simulink model "npc_controller"  (R2022a)
settings: Solver=FixedStepDiscrete  StartTime=0.0  StopTime=20  RelTol=1e-3  EnableMultiTasking=on
undefined symbols (not defined in the file): CAN_O_INT, CANA_BASE, Down, GPTRIP1SEL, GPTRIP2SEL, GPTRIP3SEL, Tsw, TZ1, TZ2, TZ3, Up, V2G_en
libraries: simulink x171, hdlsllib x90, c2802xlib x46, c2837xDlib x19, c280xlib x12, canmsglib x9, c2838xlib x8, idelinklib_common x5, c2806xlib x2, slpidlib x2, c28004xlib x2, c281xlib x2
(part 1 of 55)
settings Model: DataDictionary=param.sldd  ExtModeTrigDuration=8  Creator=The MathWorks, Inc.  LastModifiedBy=sgcesuser3
settings SolverCC: AlgebraicLoopSolver=TrustRegion  AutoInsertRateTranBlk=on  MaxZcPerStep=1
settings DataIOCC: LimitDataPoints=on  SaveFormat=Array  SaveOutput=off  SaveTime=off  ReturnWorkspaceOutputs=off
settings OptimizationCC: DefaultParameterBehavior=Inlined  MemcpyThreshold=512  ExpressionDepthLimit=2147483647  LifeSpan=1  MaxStackSize=512  EfficientTunableParamExpr=on
settings DebuggingCC: MergeDetectMultiDrivingBlocksExec=none  SolverPrmCheckMsg=warning  MultiTaskDSMMsg=none  MultiTaskCondExecSysMsg=none  FcnCallInpInsideContextMsg=warning  UnconnectedInputMsg=warning  UnconnectedOutputMsg=warning  UnconnectedLineMsg=warning  AllowSymbolicDim=off  StateNameClashWarn=warning  SFUnexpectedBacktrackingDiag=warning  SFNoUnconditionalDefaultTransitionDiag=warning  SFExecutionAtInitializationDiag=none  SFMachineParentedDataDiag=warning  ArithmeticOperatorsInVariantConditions=warning
settings HardwareCC: ProdBitPerChar=16  ProdBitPerInt=16  ProdBitPerPointer=32  ProdBitPerSizeT=32  ProdBitPerPtrDiffT=32  ProdLargestAtomicInteger=Integer  ProdLargestAtomicFloat=None  ProdWordSize=16  ProdHWDeviceType=Texas Instruments->C2000
settings ModelReferenceCC: ModelReferenceNumInstancesAllowed=Single  PropagateSignalLabelsOutOfModel=off
settings SFSimCC: SimUseLocalCustomCode=off  MATLABDynamicMemAlloc=off  CustomCodeUndefinedFunction=UseInterfaceOnly
settings RTWCC: SystemTargetFile=ert.tlc  HardwareBoard=TI Delfino F2837xS  TemplateMakefile=ert_default_tmf  GenerateReport=on  RTWUseLocalCustomCode=off  Toolchain=Texas Instruments Code Composer Studio (C2000)  BuildConfiguration=Specify  IncludeHyperlinkInReport=on  LaunchReport=on  GenerateTraceInfo=on  GenerateTraceReport=on  GenerateTraceReportSl=on  GenerateTraceReportSf=on  GenerateTraceReportEml=on  DLArmComputeVersion=19.05
settings RTWCC: CustomHeaderCode=|
  | //#include "adc.h"
  | #include "asysctl.h"
  | //#include "can.h"
  | #include "cla.h"
  | #include "cmpss.h"
  | #include "cpu.h"
  | #include "cputimer.h"
  | #include "dac.h"
  | #include "dcsm.h"
  | #include "debug.h"
  | #include "dma.h"
  | #include "ecap.h"
  | #include "emif.h"
  | #include "epwm.h"
  | #include "eqep.h"
  | #include "flash.h"
  | #include "gpio.h"
  | #include "hrpwm.h"
  | #include "i2c.h"
  | #include "interrupt.h"
  | #include "mcbsp.h"
  | #include "memcfg.h"
  | #include "pin_map.h"
  | #include "sci.h"
  | #include "sdfm.h"
  | #include "spi.h"
  | #include "sysctl.h"
  | //#include "upp.h"
  | #include "version.h"
  | #include "xbar.h"
  | //#include "clb.h"
  | //#include "clb_config.h"
settings RTWCC: CustomInclude=|
  | C:\ti\C2000\C2000Ware_4_00_00_00\driverlib\f2837xs\driverlib
  | C:\ti\C2000\C2000Ware_4_00_00_00\device_support\f2837xs\common\include
settings RTWCC: CustomSource=|
  | C:\ti\C2000\C2000Ware_4_00_00_00\driverlib\f2837xs\driverlib\cmpss.c
  | C:\ti\C2000\C2000Ware_4_00_00_00\driverlib\f2837xs\driverlib\xbar.c
  | C:\ti\C2000\C2000Ware_4_00_00_00\driverlib\f2837xs\driverlib\gpio.c
  | C:\ti\C2000\C2000Ware_4_00_00_00\driverlib\f2837xs\driverlib\clb.c
settings CodeAppCC: IgnoreCustomStorageClasses=off  CustomSymbolStrType=$N$R$M  StateflowObjectComments=on  InternalIdentifier=Classic
settings ERTTargetCC: MultiwordLength=2048  ExtModeStaticAllocSize=2048  InlinedParameterPlacement=NonHierarchical  ConvertIfToSwitch=off  SuppressUnreachableDefaultCases=off  MemSecPackage=tic2000demospkg
settings ConfigComp: CovMetricSettings=dw  CovSaveCumulativeToWorkspaceVar=on  CovSaveSingleToWorkspaceVar=on  CovExternalEMLEnable=off  CovSFcnEnable=off

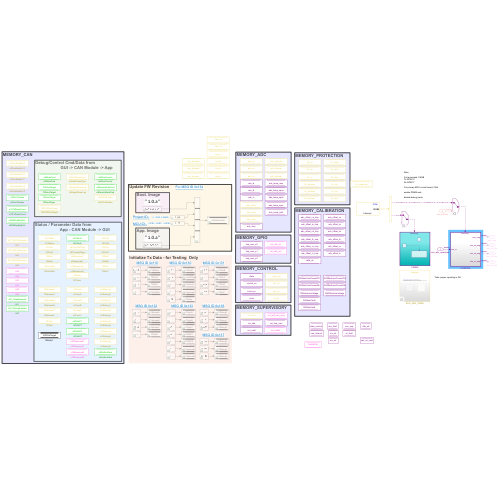
[thumbnail: Simulink's stored preview of the top-level diagram]
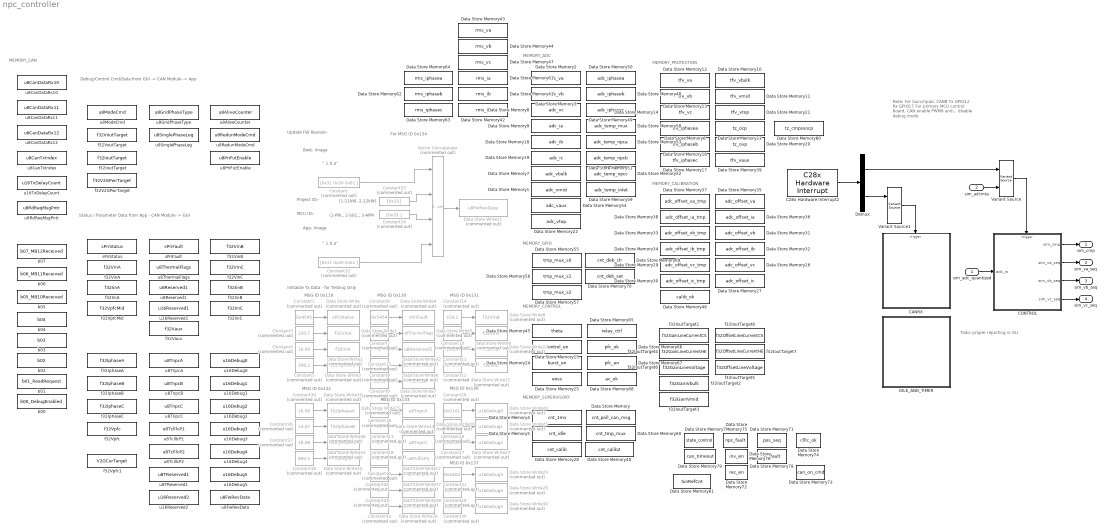
== system npc_controller ==
  note: Todo: proper reporting in GU
  note: MEMORY_CONTROL
  note: MEMORY_ADC
  note: MEMORY_CALIBRATION
  note: MEMORY_GPIO
  note: MEMORY_PROTECTION
  note: MEMORY_SUPERVISORY
  note: Boot. Image
  note: MSG ID 0x110
  note: MSG ID 0x130
  note: " 1.0.a"
  note: For MSG ID 0x134
  note: MSG ID 0x132
  note: Project ID:-
  note: MCU ID:-
  note: MSG ID 0x131
  note: " 1.0.a"
  note: MSG ID 0x133
  note: App. Image
  note: (1-11kW, 2-22kW)
  note: Debug/Control Cmd/Data from
      |                       GUI -> CAN Module -> App
  note: Update FW Revision
  note: Note:
      |
      | For launchpad, CANB
      | Tx GPIO12
      | Rx GPIO17
      |
      | For primary MCU control board, CAN
      |
      | enable PWM9 and...
      |
      | disable debug mode
  note: MEMORY_CAN
  note: Status / Parameter Data from
      |                       App - CAN Module -> GUI
  note: (1-PRI., 2-SEC., 3-APM
  note: MSG ID 0x136
  note: MSG ID 0x137
  note: Initialize Tx Data - for Testing Only
  sim_adc_quantized : Inport
  sim_adcinta : Inport  Port=2  OutputFunctionCall=on
  C28x Hardware Interrupt2 : c2000lib/Scheduling/C28x Hardware Interrupt  irqnumbers=[1 9]  pienumbers=[1 5]  irqpriorities=[30 31]  irqpreempts=[0 1]  showinput=off  dspchiptype=C280X
      settings: SourceProductBaseCode=TIC2000
  CANRX : Subsystem  TreatAsAtomicUnit=on
      settings: RTWFcnNameOpts=Use subsystem name  RTWFileNameOpts=Use subsystem name
  CONTROL : Subsystem  TreatAsAtomicUnit=on  RTWFcnName=Cla1Task1  RTWFileName=sample_cla
      settings: RTWFileNameOpts=User specified  RTWMemSecFuncInitTerm=Default  RTWMemSecFuncExecute=Default  RTWMemSecDataInternal=Default
  Constant : Constant  Commented=on  Value=[0x31 0x30 0x61 ]  OutDataTypeStr=uint8  SampleTime=-1
  Constant1 : Constant  Commented=on  Value=0x4545  OutDataTypeStr=uint16
  Constant10 : Constant  Commented=on  Value=321.2  OutDataTypeStr=single
  Constant11 : Constant  Commented=on  Value=15.09  OutDataTypeStr=single
  Constant12 : Constant  Commented=on  Value=17.09  OutDataTypeStr=single
  Constant13 : Constant  Commented=on  Value=28  OutDataTypeStr=uint8
  Constant14 : Constant  Commented=on  Value=319.2  OutDataTypeStr=single
  Constant16 : Constant  Commented=on  Value=25  OutDataTypeStr=uint8
  Constant17 : Constant  Commented=on  Value=27  OutDataTypeStr=uint8
  Constant18 : Constant  Commented=on  Value=31  OutDataTypeStr=uint8
  Constant26 : Constant  Commented=on  Value=0x0202  OutDataTypeStr=uint16
  Constant27 : Constant  Commented=on  Value=0x0303  OutDataTypeStr=uint16
  Constant28 : Constant  Commented=on  Value=0x0101  OutDataTypeStr=uint16
  Constant29 : Constant  Commented=on  Value=0x0505  OutDataTypeStr=uint16
  Constant3 : Constant  Commented=on  Value=320.7  OutDataTypeStr=single
  Constant30 : Constant  Commented=on  Value=0x0606  OutDataTypeStr=uint16
  Constant31 : Constant  Commented=on  Value=0x0404  OutDataTypeStr=uint16
  Constant32 : Constant  Commented=on  Value=[0x31 0x30 0x61 ]  OutDataTypeStr=uint8  SampleTime=-1
  Constant33 : Constant  Commented=on  Value=[0x31]  OutDataTypeStr=uint8  SampleTime=-1
  Constant34 : Constant  Commented=on  Value=[0x31 ]  OutDataTypeStr=uint8  SampleTime=-1
  Constant35 : Constant  Commented=on  Value=0  OutDataTypeStr=uint8
  Constant36 : Constant  Commented=on  Value=14.07  OutDataTypeStr=single
  Constant37 : Constant  Commented=on  Value=18.08  OutDataTypeStr=single
  Constant38 : Constant  Commented=on  Value=800.5  OutDataTypeStr=single
  Constant39 : Constant  Commented=on  Value=16.09  OutDataTypeStr=single
  Constant4 : Constant  Commented=on  Value=16.09  OutDataTypeStr=single
  Constant40 : Constant  Commented=on  Value=29  OutDataTypeStr=uint8
  Constant41 : Constant  Commented=on  Value=0  OutDataTypeStr=uint8
  Constant42 : Constant  Commented=on  Value=0  OutDataTypeStr=uint16
  Constant5 : Constant  Commented=on  Value=396.2  OutDataTypeStr=single
  Constant6 : Constant  Commented=on  Value=0x5454  OutDataTypeStr=uint16
  Constant7 : Constant  Commented=on  Value=0x0A  OutDataTypeStr=uint8
  Constant8 : Constant  Commented=on  Value=0  OutDataTypeStr=uint16
  Constant9 : Constant  Commented=on  Value=11.95  OutDataTypeStr=single
  Data Store Memory : DataStoreMemory  DataStoreName=cnt_poll_can_msg  ReadBeforeWriteMsg=warning  WriteAfterWriteMsg=warning  WriteAfterReadMsg=warning  ShowAdditionalParam=off  OutDataTypeStr=uint16
  Data Store Memory1 : DataStoreMemory  DataStoreName=adc_vmid  ReadBeforeWriteMsg=warning  WriteAfterWriteMsg=warning  WriteAfterReadMsg=warning  ShowAdditionalParam=off  OutDataTypeStr=single
  Data Store Memory10 : DataStoreMemory  DataStoreName=tfv_vbulk  ReadBeforeWriteMsg=warning  WriteAfterWriteMsg=warning  WriteAfterReadMsg=warning  ShowAdditionalParam=off  OutDataTypeStr=boolean
  Data Store Memory11 : DataStoreMemory  DataStoreName=tfv_vmid  ReadBeforeWriteMsg=warning  WriteAfterWriteMsg=warning  WriteAfterReadMsg=warning  ShowAdditionalParam=off  OutDataTypeStr=boolean
  Data Store Memory12 : DataStoreMemory  DataStoreName=tfv_va  ReadBeforeWriteMsg=warning  WriteAfterWriteMsg=warning  WriteAfterReadMsg=warning  ShowAdditionalParam=off  OutDataTypeStr=boolean
  Data Store Memory13 : DataStoreMemory  DataStoreName=tfv_vb  ReadBeforeWriteMsg=warning  WriteAfterWriteMsg=warning  WriteAfterReadMsg=warning  ShowAdditionalParam=off  OutDataTypeStr=boolean
  Data Store Memory14 : DataStoreMemory  DataStoreName=tfv_vc  ReadBeforeWriteMsg=warning  WriteAfterWriteMsg=warning  WriteAfterReadMsg=warning  ShowAdditionalParam=off  OutDataTypeStr=boolean
  Data Store Memory15 : DataStoreMemory  DataStoreName=control_en  ReadBeforeWriteMsg=warning  WriteAfterWriteMsg=warning  WriteAfterReadMsg=warning  ShowAdditionalParam=off  OutDataTypeStr=boolean
  Data Store Memory16 : DataStoreMemory  DataStoreName=tfv_iphaseb  ReadBeforeWriteMsg=warning  WriteAfterWriteMsg=warning  WriteAfterReadMsg=warning  ShowAdditionalParam=off  OutDataTypeStr=boolean
  Data Store Memory17 : DataStoreMemory  DataStoreName=tfv_iphasec  ReadBeforeWriteMsg=warning  WriteAfterWriteMsg=warning  WriteAfterReadMsg=warning  ShowAdditionalParam=off  OutDataTypeStr=boolean
  Data Store Memory18 : DataStoreMemory  DataStoreName=adc_ib  ReadBeforeWriteMsg=warning  WriteAfterWriteMsg=warning  WriteAfterReadMsg=warning  ShowAdditionalParam=off  OutDataTypeStr=single
  Data Store Memory19 : DataStoreMemory  DataStoreName=adc_ic  ReadBeforeWriteMsg=warning  WriteAfterWriteMsg=warning  WriteAfterReadMsg=warning  ShowAdditionalParam=off  OutDataTypeStr=single
  Data Store Memory2 : DataStoreMemory  DataStoreName=adc_va  ReadBeforeWriteMsg=warning  WriteAfterWriteMsg=warning  WriteAfterReadMsg=warning  ShowAdditionalParam=off  OutDataTypeStr=single
  Data Store Memory20 : DataStoreMemory  DataStoreName=tz_ovp  ReadBeforeWriteMsg=warning  WriteAfterWriteMsg=warning  WriteAfterReadMsg=warning  ShowAdditionalParam=off  OutDataTypeStr=uint16
  Data Store Memory21 : DataStoreMemory  DataStoreName=tfv_vtop  ReadBeforeWriteMsg=warning  WriteAfterWriteMsg=warning  WriteAfterReadMsg=warning  ShowAdditionalParam=off  OutDataTypeStr=boolean
  Data Store Memory22 : DataStoreMemory  DataStoreName=adc_vtop  ReadBeforeWriteMsg=warning  WriteAfterWriteMsg=warning  WriteAfterReadMsg=warning  InitialValue=13  ShowAdditionalParam=off  OutDataTypeStr=uint16
  Data Store Memory23 : DataStoreMemory  DataStoreName=tz_ocp  ReadBeforeWriteMsg=warning  WriteAfterWriteMsg=warning  WriteAfterReadMsg=warning  ShowAdditionalParam=off  OutDataTypeStr=uint16
  Data Store Memory24 : DataStoreMemory  DataStoreName=burst_en  ReadBeforeWriteMsg=warning  WriteAfterWriteMsg=warning  WriteAfterReadMsg=warning  ShowAdditionalParam=off  OutDataTypeStr=boolean
  Data Store Memory25 : DataStoreMemory  DataStoreName=eoss  ReadBeforeWriteMsg=warning  WriteAfterWriteMsg=warning  WriteAfterReadMsg=warning  ShowAdditionalParam=off  OutDataTypeStr=boolean
  Data Store Memory26 : DataStoreMemory  DataStoreName=adc_offset_vc  ReadBeforeWriteMsg=warning  WriteAfterWriteMsg=warning  WriteAfterReadMsg=warning  ShowAdditionalParam=off  OutDataTypeStr=single
  Data Store Memory27 : DataStoreMemory  DataStoreName=adc_offset_ic  ReadBeforeWriteMsg=warning  WriteAfterWriteMsg=warning  WriteAfterReadMsg=warning  ShowAdditionalParam=off  OutDataTypeStr=single
  Data Store Memory28 : DataStoreMemory  DataStoreName=cnt_calib  ReadBeforeWriteMsg=warning  WriteAfterWriteMsg=warning  WriteAfterReadMsg=warning  InitialValue=1  ShowAdditionalParam=off  OutDataTypeStr=uint16
  Data Store Memory29 : DataStoreMemory  DataStoreName=adc_offset_vc_tmp  ReadBeforeWriteMsg=warning  WriteAfterWriteMsg=warning  WriteAfterReadMsg=warning  ShowAdditionalParam=off  OutDataTypeStr=single
  Data Store Memory3 : DataStoreMemory  DataStoreName=adc_vb  ReadBeforeWriteMsg=warning  WriteAfterWriteMsg=warning  WriteAfterReadMsg=warning  ShowAdditionalParam=off  OutDataTypeStr=single
  Data Store Memory30 : DataStoreMemory  DataStoreName=adc_offset_ic_tmp  ReadBeforeWriteMsg=warning  WriteAfterWriteMsg=warning  WriteAfterReadMsg=warning  ShowAdditionalParam=off  OutDataTypeStr=single
  Data Store Memory31 : DataStoreMemory  DataStoreName=adc_offset_vb  ReadBeforeWriteMsg=warning  WriteAfterWriteMsg=warning  WriteAfterReadMsg=warning  ShowAdditionalParam=off  OutDataTypeStr=single
  Data Store Memory32 : DataStoreMemory  DataStoreName=adc_offset_ib  ReadBeforeWriteMsg=warning  WriteAfterWriteMsg=warning  WriteAfterReadMsg=warning  ShowAdditionalParam=off  OutDataTypeStr=single
  Data Store Memory33 : DataStoreMemory  DataStoreName=adc_offset_vb_tmp  ReadBeforeWriteMsg=warning  WriteAfterWriteMsg=warning  WriteAfterReadMsg=warning  ShowAdditionalParam=off  OutDataTypeStr=single
  Data Store Memory34 : DataStoreMemory  DataStoreName=adc_offset_ib_tmp  ReadBeforeWriteMsg=warning  WriteAfterWriteMsg=warning  WriteAfterReadMsg=warning  ShowAdditionalParam=off  OutDataTypeStr=single
  Data Store Memory35 : DataStoreMemory  DataStoreName=adc_offset_va  ReadBeforeWriteMsg=warning  WriteAfterWriteMsg=warning  WriteAfterReadMsg=warning  ShowAdditionalParam=off  OutDataTypeStr=single
  Data Store Memory36 : DataStoreMemory  DataStoreName=adc_offset_ia  ReadBeforeWriteMsg=warning  WriteAfterWriteMsg=warning  WriteAfterReadMsg=warning  ShowAdditionalParam=off  OutDataTypeStr=single
  Data Store Memory37 : DataStoreMemory  DataStoreName=adc_offset_va_tmp  ReadBeforeWriteMsg=warning  WriteAfterWriteMsg=warning  WriteAfterReadMsg=warning  ShowAdditionalParam=off  OutDataTypeStr=single
  Data Store Memory38 : DataStoreMemory  DataStoreName=adc_offset_ia_tmp  ReadBeforeWriteMsg=warning  WriteAfterWriteMsg=warning  WriteAfterReadMsg=warning  ShowAdditionalParam=off  OutDataTypeStr=single
  Data Store Memory39 : DataStoreMemory  DataStoreName=tfv_vaux  ReadBeforeWriteMsg=warning  WriteAfterWriteMsg=warning  WriteAfterReadMsg=warning  ShowAdditionalParam=off  OutDataTypeStr=boolean
  Data Store Memory4 : DataStoreMemory  DataStoreName=cnt_1ms  ReadBeforeWriteMsg=warning  WriteAfterWriteMsg=warning  WriteAfterReadMsg=warning  ShowAdditionalParam=off  OutDataTypeStr=uint16
  Data Store Memory40 : DataStoreMemory  DataStoreName=cnt_calib2  ReadBeforeWriteMsg=warning  WriteAfterWriteMsg=warning  WriteAfterReadMsg=warning  InitialValue=1  ShowAdditionalParam=off  OutDataTypeStr=uint16
  Data Store Memory41 : DataStoreMemory  DataStoreName=rms_ib  ReadBeforeWriteMsg=warning  WriteAfterWriteMsg=warning  WriteAfterReadMsg=warning  ShowAdditionalParam=off  OutDataTypeStr=single
  Data Store Memory42 : DataStoreMemory  DataStoreName=rms_ic  ReadBeforeWriteMsg=warning  WriteAfterWriteMsg=warning  WriteAfterReadMsg=warning  ShowAdditionalParam=off  OutDataTypeStr=single
  Data Store Memory43 : DataStoreMemory  DataStoreName=rms_va  ReadBeforeWriteMsg=warning  WriteAfterWriteMsg=warning  WriteAfterReadMsg=warning  ShowAdditionalParam=off  OutDataTypeStr=single
  Data Store Memory44 : DataStoreMemory  DataStoreName=rms_vb  ReadBeforeWriteMsg=warning  WriteAfterWriteMsg=warning  WriteAfterReadMsg=warning  ShowAdditionalParam=off  OutDataTypeStr=single
  Data Store Memory45 : DataStoreMemory  DataStoreName=theta  ReadBeforeWriteMsg=warning  WriteAfterWriteMsg=warning  WriteAfterReadMsg=warning  ShowAdditionalParam=off  OutDataTypeStr=uint16
  Data Store Memory46 : DataStoreMemory  DataStoreName=calib_ok  ReadBeforeWriteMsg=warning  WriteAfterWriteMsg=warning  WriteAfterReadMsg=warning  ShowAdditionalParam=off  OutDataTypeStr=boolean
  Data Store Memory47 : DataStoreMemory  DataStoreName=rms_vc  ReadBeforeWriteMsg=warning  WriteAfterWriteMsg=warning  WriteAfterReadMsg=warning  ShowAdditionalParam=off  OutDataTypeStr=single
  Data Store Memory48 : DataStoreMemory  DataStoreName=adc_iphaseb  ReadBeforeWriteMsg=warning  WriteAfterWriteMsg=warning  WriteAfterReadMsg=warning  ShowAdditionalParam=off  OutDataTypeStr=single
  Data Store Memory49 : DataStoreMemory  DataStoreName=adc_iphasec  ReadBeforeWriteMsg=warning  WriteAfterWriteMsg=warning  WriteAfterReadMsg=warning  ShowAdditionalParam=off  OutDataTypeStr=single
  Data Store Memory5 : DataStoreMemory  DataStoreName=cnt_idle  ReadBeforeWriteMsg=warning  WriteAfterWriteMsg=warning  WriteAfterReadMsg=warning  ShowAdditionalParam=off  OutDataTypeStr=uint16
  Data Store Memory50 : DataStoreMemory  DataStoreName=adc_iphasea  ReadBeforeWriteMsg=warning  WriteAfterWriteMsg=warning  WriteAfterReadMsg=warning  ShowAdditionalParam=off  OutDataTypeStr=single
  Data Store Memory51 : DataStoreMemory  DataStoreName=adc_temp_npcb  ReadBeforeWriteMsg=warning  WriteAfterWriteMsg=warning  WriteAfterReadMsg=warning  ShowAdditionalParam=off  OutDataTypeStr=single
  Data Store Memory52 : DataStoreMemory  DataStoreName=adc_temp_npcc  ReadBeforeWriteMsg=warning  WriteAfterWriteMsg=warning  WriteAfterReadMsg=warning  ShowAdditionalParam=off  OutDataTypeStr=single
  Data Store Memory53 : DataStoreMemory  DataStoreName=adc_temp_npca  ReadBeforeWriteMsg=warning  WriteAfterWriteMsg=warning  WriteAfterReadMsg=warning  ShowAdditionalParam=off  OutDataTypeStr=single
  Data Store Memory54 : DataStoreMemory  DataStoreName=adc_vaux  ReadBeforeWriteMsg=warning  WriteAfterWriteMsg=warning  WriteAfterReadMsg=warning  ShowAdditionalParam=off  OutDataTypeStr=single
  Data Store Memory55 : DataStoreMemory  DataStoreName=tmp_mux_s0  ReadBeforeWriteMsg=warning  WriteAfterWriteMsg=warning  WriteAfterReadMsg=warning  InitialValue=false  ShowAdditionalParam=off  OutDataTypeStr=boolean
  Data Store Memory56 : DataStoreMemory  DataStoreName=tmp_mux_s1  ReadBeforeWriteMsg=warning  WriteAfterWriteMsg=warning  WriteAfterReadMsg=warning  InitialValue=false  ShowAdditionalParam=off  OutDataTypeStr=boolean
  Data Store Memory57 : DataStoreMemory  DataStoreName=tmp_mux_s2  ReadBeforeWriteMsg=warning  WriteAfterWriteMsg=warning  WriteAfterReadMsg=warning  InitialValue=false  ShowAdditionalParam=off  OutDataTypeStr=boolean
  Data Store Memory58 : DataStoreMemory  DataStoreName=adc_temp_mux  ReadBeforeWriteMsg=warning  WriteAfterWriteMsg=warning  WriteAfterReadMsg=warning  ShowAdditionalParam=off  OutDataTypeStr=single
  Data Store Memory59 : DataStoreMemory  DataStoreName=adc_temp_inlet  ReadBeforeWriteMsg=warning  WriteAfterWriteMsg=warning  WriteAfterReadMsg=warning  ShowAdditionalParam=off  OutDataTypeStr=single
  Data Store Memory6 : DataStoreMemory  DataStoreName=tfv_iphasea  ReadBeforeWriteMsg=warning  WriteAfterWriteMsg=warning  WriteAfterReadMsg=warning  ShowAdditionalParam=off  OutDataTypeStr=boolean
  Data Store Memory60 : DataStoreMemory  DataStoreName=cnt_tmp_mux  ReadBeforeWriteMsg=warning  WriteAfterWriteMsg=warning  WriteAfterReadMsg=warning  ShowAdditionalParam=off  OutDataTypeStr=uint16
  Data Store Memory61 : DataStoreMemory  DataStoreName=rms_ia  ReadBeforeWriteMsg=warning  WriteAfterWriteMsg=warning  WriteAfterReadMsg=warning  ShowAdditionalParam=off  OutDataTypeStr=single
  Data Store Memory62 : DataStoreMemory  DataStoreName=rms_iphaseb  ReadBeforeWriteMsg=warning  WriteAfterWriteMsg=warning  WriteAfterReadMsg=warning  ShowAdditionalParam=off  OutDataTypeStr=single
  Data Store Memory63 : DataStoreMemory  DataStoreName=rms_iphasec  ReadBeforeWriteMsg=warning  WriteAfterWriteMsg=warning  WriteAfterReadMsg=warning  ShowAdditionalParam=off  OutDataTypeStr=single
  Data Store Memory64 : DataStoreMemory  DataStoreName=rms_iphasea  ReadBeforeWriteMsg=warning  WriteAfterWriteMsg=warning  WriteAfterReadMsg=warning  ShowAdditionalParam=off  OutDataTypeStr=single
  Data Store Memory65 : DataStoreMemory  DataStoreName=relay_ctrl  ReadBeforeWriteMsg=warning  WriteAfterWriteMsg=warning  WriteAfterReadMsg=warning  ShowAdditionalParam=off  OutDataTypeStr=boolean
  Data Store Memory66 : DataStoreMemory  DataStoreName=pfc_ok  ReadBeforeWriteMsg=warning  WriteAfterWriteMsg=warning  WriteAfterReadMsg=warning  ShowAdditionalParam=off  OutDataTypeStr=boolean
  Data Store Memory67 : DataStoreMemory  DataStoreName=pfc_en  ReadBeforeWriteMsg=warning  WriteAfterWriteMsg=warning  WriteAfterReadMsg=warning  ShowAdditionalParam=off  OutDataTypeStr=boolean
  Data Store Memory68 : DataStoreMemory  DataStoreName=ac_ok  ReadBeforeWriteMsg=warning  WriteAfterWriteMsg=warning  WriteAfterReadMsg=warning  ShowAdditionalParam=off  OutDataTypeStr=boolean
  Data Store Memory69 : DataStoreMemory  DataStoreName=cnt_deb_clr  WriteAfterWriteMsg=warning  ShowAdditionalParam=off  OutDataTypeStr=uint16
  Data Store Memory7 : DataStoreMemory  DataStoreName=adc_vbulk  ReadBeforeWriteMsg=warning  WriteAfterWriteMsg=warning  WriteAfterReadMsg=warning  ShowAdditionalParam=off  OutDataTypeStr=single
  Data Store Memory70 : DataStoreMemory  DataStoreName=cnt_deb_set  WriteAfterWriteMsg=warning  ShowAdditionalParam=off  OutDataTypeStr=uint16
  Data Store Memory71 : DataStoreMemory  DataStoreName=pos_seq  WriteAfterWriteMsg=warning  ShowAdditionalParam=off
  Data Store Memory72 : DataStoreMemory  DataStoreName=rec_en  WriteAfterWriteMsg=warning  ShowAdditionalParam=off
  Data Store Memory73 : DataStoreMemory  DataStoreName=can_on_cmd  WriteAfterWriteMsg=warning  ShowAdditionalParam=off
  Data Store Memory74 : DataStoreMemory  DataStoreName=clllc_ok  WriteAfterWriteMsg=warning  ShowAdditionalParam=off
  Data Store Memory75 : DataStoreMemory  DataStoreName=npc_fault  WriteAfterWriteMsg=warning  ShowAdditionalParam=off
  Data Store Memory76 : DataStoreMemory  DataStoreName=inv_en  WriteAfterWriteMsg=warning  ShowAdditionalParam=off
  Data Store Memory77 : DataStoreMemory  DataStoreName=state_control  WriteAfterWriteMsg=warning  ShowAdditionalParam=off
  Data Store Memory78 : DataStoreMemory  DataStoreName=ot_fault  WriteAfterWriteMsg=warning  ShowAdditionalParam=off
  Data Store Memory79 : DataStoreMemory  DataStoreName=can_timeout  WriteAfterWriteMsg=warning  ShowAdditionalParam=off
  Data Store Memory8 : DataStoreMemory  DataStoreName=adc_vc  ReadBeforeWriteMsg=warning  WriteAfterWriteMsg=warning  WriteAfterReadMsg=warning  ShowAdditionalParam=off  OutDataTypeStr=single
  Data Store Memory80 : DataStoreMemory  DataStoreName=tz_cmpssocp  ReadBeforeWriteMsg=warning  WriteAfterWriteMsg=warning  WriteAfterReadMsg=warning  ShowAdditionalParam=off  OutDataTypeStr=uint16
  Data Store Memory81 : DataStoreMemory  DataStoreName=SinRefCnt  WriteAfterWriteMsg=warning  ShowAdditionalParam=off  OutDataTypeStr=single
  Data Store Memory9 : DataStoreMemory  DataStoreName=adc_ia  ReadBeforeWriteMsg=warning  WriteAfterWriteMsg=warning  WriteAfterReadMsg=warning  ShowAdditionalParam=off  OutDataTypeStr=single
  Data Store Write : DataStoreWrite  Commented=on  DataStoreName=sPriStatus  IndexOptions=Index vector (dialog)  Indices=1  OutputSizes=1
  Data Store Write1 : DataStoreWrite  Commented=on  DataStoreName=f32VinA  IndexOptions=Index vector (dialog)  Indices=1  OutputSizes=1
  Data Store Write10 : DataStoreWrite  Commented=on  DataStoreName=f32IinB  IndexOptions=Index vector (dialog)  Indices=1  OutputSizes=1
  Data Store Write11 : DataStoreWrite  Commented=on  DataStoreName=f32IinC  IndexOptions=Index vector (dialog)  Indices=1  OutputSizes=1
  Data Store Write14 : DataStoreWrite  Commented=on  DataStoreName=u8TnpcC  IndexOptions=Index vector (dialog)  Indices=1  OutputSizes=1
  Data Store Write15 : DataStoreWrite  Commented=on  DataStoreName=u8TnpcA  IndexOptions=Index vector (dialog)  Indices=1  OutputSizes=1
  Data Store Write16 : DataStoreWrite  Commented=on  DataStoreName=u8TnpcB  IndexOptions=Index vector (dialog)  Indices=1  OutputSizes=1
  Data Store Write17 : DataStoreWrite  Commented=on  DataStoreName=u8TclllcP1  IndexOptions=Index vector (dialog)  Indices=1  OutputSizes=1
  Data Store Write2 : DataStoreWrite  Commented=on  DataStoreName=f32IinA  IndexOptions=Index vector (dialog)  Indices=1  OutputSizes=1
  Data Store Write25 : DataStoreWrite  Commented=on  DataStoreName=u16Debug1  IndexOptions=Index vector (dialog)  Indices=1  OutputSizes=1
  Data Store Write26 : DataStoreWrite  Commented=on  DataStoreName=u16Debug0  IndexOptions=Index vector (dialog)  Indices=1  OutputSizes=1
  Data Store Write27 : DataStoreWrite  Commented=on  DataStoreName=u16Debug2  IndexOptions=Index vector (dialog)  Indices=1  OutputSizes=1
  Data Store Write28 : DataStoreWrite  Commented=on  DataStoreName=u16Debug4  IndexOptions=Index vector (dialog)  Indices=1  OutputSizes=1
  Data Store Write29 : DataStoreWrite  Commented=on  DataStoreName=u16Debug3  IndexOptions=Index vector (dialog)  Indices=1  OutputSizes=1
  Data Store Write3 : DataStoreWrite  Commented=on  DataStoreName=f32VpfcMid  IndexOptions=Index vector (dialog)  Indices=1  OutputSizes=1
  Data Store Write30 : DataStoreWrite  Commented=on  DataStoreName=u16Debug5  IndexOptions=Index vector (dialog)  Indices=1  OutputSizes=1
  Data Store Write31 : DataStoreWrite  Commented=on  DataStoreName=u8FwRevData  IndexOptions=Index vector (dialog)  Indices=1  OutputSizes=1
  Data Store Write32 : DataStoreWrite  Commented=on  DataStoreName=u8Reserved1  IndexOptions=Index vector (dialog)  Indices=1  OutputSizes=1
  Data Store Write33 : DataStoreWrite  Commented=on  DataStoreName=f32IphaseC  IndexOptions=Index vector (dialog)  Indices=1  OutputSizes=1
  Data Store Write34 : DataStoreWrite  Commented=on  DataStoreName=f32Vpfc  IndexOptions=Index vector (dialog)  Indices=1  OutputSizes=1
  Data Store Write35 : DataStoreWrite  Commented=on  DataStoreName=f32IphaseA  IndexOptions=Index vector (dialog)  Indices=1  OutputSizes=1
  Data Store Write36 : DataStoreWrite  Commented=on  DataStoreName=f32IphaseB  IndexOptions=Index vector (dialog)  Indices=1  OutputSizes=1
  Data Store Write37 : DataStoreWrite  Commented=on  DataStoreName=u8TclllcP2  IndexOptions=Index vector (dialog)  Indices=1  OutputSizes=1
  Data Store Write38 : DataStoreWrite  Commented=on  DataStoreName=u8TReserved1  IndexOptions=Index vector (dialog)  Indices=1  OutputSizes=1
  Data Store Write39 : DataStoreWrite  Commented=on  DataStoreName=u16Reserved2  IndexOptions=Index vector (dialog)  Indices=1  OutputSizes=1
  Data Store Write4 : DataStoreWrite  Commented=on  DataStoreName=sPriFault  IndexOptions=Index vector (dialog)  Indices=1  OutputSizes=1
  Data Store Write5 : DataStoreWrite  Commented=on  DataStoreName=u8ThermalFlags  IndexOptions=Index vector (dialog)  Indices=1  OutputSizes=1
  Data Store Write6 : DataStoreWrite  Commented=on  DataStoreName=u16Reserved1  IndexOptions=Index vector (dialog)  Indices=1  OutputSizes=1
  Data Store Write7 : DataStoreWrite  Commented=on  DataStoreName=f32Vaux  IndexOptions=Index vector (dialog)  Indices=1  OutputSizes=1
  Data Store Write8 : DataStoreWrite  Commented=on  DataStoreName=f32VinB  IndexOptions=Index vector (dialog)  Indices=1  OutputSizes=1
  Data Store Write9 : DataStoreWrite  Commented=on  DataStoreName=f32VinC  IndexOptions=Index vector (dialog)  Indices=1  OutputSizes=1
  Demux : Demux  Outputs=2
  IDLE_AND_TIMER : Subsystem  Variant=on
  Variant Source : VariantSource  OutputFunctionCall=on
  Variant Source1 : VariantSource
  Vector Concatenate : Concatenate  Commented=on  NumInputs=4
  b00 : DataStoreMemory  DataStoreName=b00_DebugEnabled  ReadBeforeWriteMsg=warning  WriteAfterWriteMsg=warning  WriteAfterReadMsg=warning  ShowAdditionalParam=off  OutDataTypeStr=boolean
  b01 : DataStoreMemory  DataStoreName=b01_ReadRequest  ReadBeforeWriteMsg=warning  WriteAfterWriteMsg=warning  WriteAfterReadMsg=warning  ShowAdditionalParam=off  OutDataTypeStr=boolean
  b02 : DataStoreMemory  DataStoreName=b02  ReadBeforeWriteMsg=warning  WriteAfterWriteMsg=warning  WriteAfterReadMsg=warning  ShowAdditionalParam=off  OutDataTypeStr=boolean
  b03 : DataStoreMemory  DataStoreName=b03  ReadBeforeWriteMsg=warning  WriteAfterWriteMsg=warning  WriteAfterReadMsg=warning  ShowAdditionalParam=off  OutDataTypeStr=boolean
  b04 : DataStoreMemory  DataStoreName=b04  ReadBeforeWriteMsg=warning  WriteAfterWriteMsg=warning  WriteAfterReadMsg=warning  ShowAdditionalParam=off  OutDataTypeStr=boolean
  b05 : DataStoreMemory  DataStoreName=b05_MB10Received  ReadBeforeWriteMsg=warning  WriteAfterWriteMsg=warning  WriteAfterReadMsg=warning  ShowAdditionalParam=off  OutDataTypeStr=boolean
  b06 : DataStoreMemory  DataStoreName=b06_MB11Received  ReadBeforeWriteMsg=warning  WriteAfterWriteMsg=warning  WriteAfterReadMsg=warning  ShowAdditionalParam=off  OutDataTypeStr=boolean
  b07 : DataStoreMemory  DataStoreName=b07_MB12Received  ReadBeforeWriteMsg=warning  WriteAfterWriteMsg=warning  WriteAfterReadMsg=warning  ShowAdditionalParam=off  OutDataTypeStr=boolean
  f32IinA : DataStoreMemory  DataStoreName=f32IinA  ReadBeforeWriteMsg=warning  WriteAfterWriteMsg=warning  WriteAfterReadMsg=warning  ShowAdditionalParam=off  OutDataTypeStr=single
  f32IinB : DataStoreMemory  DataStoreName=f32IinB  ReadBeforeWriteMsg=warning  WriteAfterWriteMsg=warning  WriteAfterReadMsg=warning  ShowAdditionalParam=off  OutDataTypeStr=single
  f32IinC : DataStoreMemory  DataStoreName=f32IinC  ReadBeforeWriteMsg=warning  WriteAfterWriteMsg=warning  WriteAfterReadMsg=warning  ShowAdditionalParam=off  OutDataTypeStr=single
  f32IoutTarget : DataStoreMemory  DataStoreName=f32IoutTarget  ReadBeforeWriteMsg=warning  WriteAfterWriteMsg=warning  WriteAfterReadMsg=warning  InitialValue=0.0  ShowAdditionalParam=off  OutDataTypeStr=single
  f32IoutTarget1 : DataStoreMemory  DataStoreName=f32GainLineCurrentCS  ReadBeforeWriteMsg=warning  WriteAfterWriteMsg=warning  WriteAfterReadMsg=warning  InitialValue=(3.3/4095)*(1/0.019523)  ShowAdditionalParam=off  OutDataTypeStr=single
  f32IoutTarget2 : DataStoreMemory  DataStoreName=f32GainVbulk  ReadBeforeWriteMsg=warning  WriteAfterWriteMsg=warning  WriteAfterReadMsg=warning  InitialValue=(3.3/4095)*(1/0.00356)  ShowAdditionalParam=off  OutDataTypeStr=single
  f32IoutTarget3 : DataStoreMemory  DataStoreName=f32GainVmid  ReadBeforeWriteMsg=warning  WriteAfterWriteMsg=warning  WriteAfterReadMsg=warning  InitialValue=(3.3/4095)*(1/0.00633)  ShowAdditionalParam=off  OutDataTypeStr=single
  f32IoutTarget4 : DataStoreMemory  DataStoreName=f32GainLineCurrentHE  ReadBeforeWriteMsg=warning  WriteAfterWriteMsg=warning  WriteAfterReadMsg=warning  InitialValue=(3.3/4095)*(1/0.02)  ShowAdditionalParam=off  OutDataTypeStr=single
  f32IoutTarget5 : DataStoreMemory  DataStoreName=f32OffsetLineVoltage  ReadBeforeWriteMsg=warning  WriteAfterWriteMsg=warning  WriteAfterReadMsg=warning  ShowAdditionalParam=off  OutDataTypeStr=single
  f32IoutTarget6 : DataStoreMemory  DataStoreName=f32GainLineVoltage  ReadBeforeWriteMsg=warning  WriteAfterWriteMsg=warning  WriteAfterReadMsg=warning  InitialValue=(3.3/4095)*(1/0.001799)  ShowAdditionalParam=off  OutDataTypeStr=single
  f32IoutTarget7 : DataStoreMemory  DataStoreName=f32OffsetLineCurrentHE  ReadBeforeWriteMsg=warning  WriteAfterWriteMsg=warning  WriteAfterReadMsg=warning  ShowAdditionalParam=off  OutDataTypeStr=single
  f32IoutTarget8 : DataStoreMemory  DataStoreName=f32OffsetLineCurrentCS  ReadBeforeWriteMsg=warning  WriteAfterWriteMsg=warning  WriteAfterReadMsg=warning  ShowAdditionalParam=off  OutDataTypeStr=single
  f32IphaseA : DataStoreMemory  DataStoreName=f32IphaseA  ReadBeforeWriteMsg=warning  WriteAfterWriteMsg=warning  WriteAfterReadMsg=warning  ShowAdditionalParam=off  OutDataTypeStr=single
  f32IphaseB : DataStoreMemory  DataStoreName=f32IphaseB  ReadBeforeWriteMsg=warning  WriteAfterWriteMsg=warning  WriteAfterReadMsg=warning  ShowAdditionalParam=off  OutDataTypeStr=single
  f32IphaseC : DataStoreMemory  DataStoreName=f32IphaseC  ReadBeforeWriteMsg=warning  WriteAfterWriteMsg=warning  WriteAfterReadMsg=warning  ShowAdditionalParam=off  OutDataTypeStr=single
  f32V2GPwrTarget : DataStoreMemory  DataStoreName=f32V2GPwrTarget  ReadBeforeWriteMsg=warning  WriteAfterWriteMsg=warning  WriteAfterReadMsg=warning  InitialValue=0.0  ShowAdditionalParam=off  OutDataTypeStr=single
  f32Vaux : DataStoreMemory  DataStoreName=f32Vaux  ReadBeforeWriteMsg=warning  WriteAfterWriteMsg=warning  WriteAfterReadMsg=warning  ShowAdditionalParam=off  OutDataTypeStr=single
  f32VinA : DataStoreMemory  DataStoreName=f32VinA  ReadBeforeWriteMsg=warning  WriteAfterWriteMsg=warning  WriteAfterReadMsg=warning  ShowAdditionalParam=off  OutDataTypeStr=single
  f32VinB : DataStoreMemory  DataStoreName=f32VinB  ReadBeforeWriteMsg=warning  WriteAfterWriteMsg=warning  WriteAfterReadMsg=warning  ShowAdditionalParam=off  OutDataTypeStr=single
  f32VinC : DataStoreMemory  DataStoreName=f32VinC  ReadBeforeWriteMsg=warning  WriteAfterWriteMsg=warning  WriteAfterReadMsg=warning  ShowAdditionalParam=off  OutDataTypeStr=single
  f32VoutTarget : DataStoreMemory  DataStoreName=f32VoutTarget  ReadBeforeWriteMsg=warning  WriteAfterWriteMsg=warning  WriteAfterReadMsg=warning  InitialValue=0.0  ShowAdditionalParam=off  OutDataTypeStr=single
  f32Vpfc : DataStoreMemory  DataStoreName=f32Vpfc  ReadBeforeWriteMsg=warning  WriteAfterWriteMsg=warning  WriteAfterReadMsg=warning  ShowAdditionalParam=off  OutDataTypeStr=single
  f32Vpfc1 : DataStoreMemory  DataStoreName=V2GCurTarget  ReadBeforeWriteMsg=warning  WriteAfterWriteMsg=warning  WriteAfterReadMsg=warning  ShowAdditionalParam=off  OutDataTypeStr=single
  f32VpfcMid : DataStoreMemory  DataStoreName=f32VpfcMid  ReadBeforeWriteMsg=warning  WriteAfterWriteMsg=warning  WriteAfterReadMsg=warning  ShowAdditionalParam=off  OutDataTypeStr=single
  sPriFault : DataStoreMemory  DataStoreName=sPriFault  ReadBeforeWriteMsg=warning  WriteAfterWriteMsg=warning  WriteAfterReadMsg=warning  ShowAdditionalParam=off  OutDataTypeStr=uint16
  sPriStatus : DataStoreMemory  DataStoreName=sPriStatus  ReadBeforeWriteMsg=warning  WriteAfterWriteMsg=warning  WriteAfterReadMsg=warning  ShowAdditionalParam=off  OutDataTypeStr=uint16
  u16Debug0 : DataStoreMemory  DataStoreName=u16Debug0  ReadBeforeWriteMsg=warning  WriteAfterWriteMsg=warning  WriteAfterReadMsg=warning  ShowAdditionalParam=off  OutDataTypeStr=uint16
  u16Debug1 : DataStoreMemory  DataStoreName=u16Debug1  ReadBeforeWriteMsg=warning  WriteAfterWriteMsg=warning  WriteAfterReadMsg=warning  ShowAdditionalParam=off  OutDataTypeStr=uint16
  u16Debug2 : DataStoreMemory  DataStoreName=u16Debug2  ReadBeforeWriteMsg=warning  WriteAfterWriteMsg=warning  WriteAfterReadMsg=warning  ShowAdditionalParam=off  OutDataTypeStr=uint16
  u16Debug3 : DataStoreMemory  DataStoreName=u16Debug3  ReadBeforeWriteMsg=warning  WriteAfterWriteMsg=warning  WriteAfterReadMsg=warning  ShowAdditionalParam=off  OutDataTypeStr=uint16
  u16Debug4 : DataStoreMemory  DataStoreName=u16Debug4  ReadBeforeWriteMsg=warning  WriteAfterWriteMsg=warning  WriteAfterReadMsg=warning  ShowAdditionalParam=off  OutDataTypeStr=uint16
  u16Debug5 : DataStoreMemory  DataStoreName=u16Debug5  ReadBeforeWriteMsg=warning  WriteAfterWriteMsg=warning  WriteAfterReadMsg=warning  ShowAdditionalParam=off  OutDataTypeStr=uint16
  u16Reserved1 : DataStoreMemory  DataStoreName=u16Reserved1  ReadBeforeWriteMsg=warning  WriteAfterWriteMsg=warning  WriteAfterReadMsg=warning  ShowAdditionalParam=off  OutDataTypeStr=uint16
  u16Reserved2 : DataStoreMemory  DataStoreName=u16Reserved2  ReadBeforeWriteMsg=warning  WriteAfterWriteMsg=warning  WriteAfterReadMsg=warning  ShowAdditionalParam=off  OutDataTypeStr=uint16
  u16TxDelayCount : DataStoreMemory  DataStoreName=u16TxDelayCount  ReadBeforeWriteMsg=warning  WriteAfterWriteMsg=warning  WriteAfterReadMsg=warning  ShowAdditionalParam=off  OutDataTypeStr=uint16
  u8AliveCounter : DataStoreMemory  DataStoreName=u8AliveCounter  ReadBeforeWriteMsg=warning  WriteAfterWriteMsg=warning  WriteAfterReadMsg=warning  ShowAdditionalParam=off  OutDataTypeStr=uint8
  u8CanDataRx10 : DataStoreMemory  DataStoreName=u8CanDataRx10  ReadBeforeWriteMsg=warning  WriteAfterWriteMsg=warning  WriteAfterReadMsg=warning  InitialValue=[0 0 0 0 0 0 0 0]  ShowAdditionalParam=off  OutDataTypeStr=uint8  Dimensions=[8 1]
  u8CanDataRx11 : DataStoreMemory  DataStoreName=u8CanDataRx11  ReadBeforeWriteMsg=warning  WriteAfterWriteMsg=warning  WriteAfterReadMsg=warning  InitialValue=[0 0 0 0 0 0 0 0]  ShowAdditionalParam=off  OutDataTypeStr=uint8  Dimensions=[8 1]
  u8CanDataRx12 : DataStoreMemory  DataStoreName=u8CanDataRx12  ReadBeforeWriteMsg=warning  WriteAfterWriteMsg=warning  WriteAfterReadMsg=warning  InitialValue=[0 0 0 0 0 0 0 0]  ShowAdditionalParam=off  OutDataTypeStr=uint8  Dimensions=[8 1]
  u8CanTxIndex : DataStoreMemory  DataStoreName=u8CanTxIndex  ReadBeforeWriteMsg=warning  WriteAfterWriteMsg=warning  WriteAfterReadMsg=warning  ShowAdditionalParam=off  OutDataTypeStr=uint8
  u8FwRevData : DataStoreMemory  DataStoreName=u8FwRevData  ReadBeforeWriteMsg=warning  WriteAfterWriteMsg=warning  WriteAfterReadMsg=warning  InitialValue=[0 0 0 0 0 0 0 0]  ShowAdditionalParam=off  OutDataTypeStr=uint8  Dimensions=[8 1]
  u8GridPhaseType : DataStoreMemory  DataStoreName=u8GridPhaseType  ReadBeforeWriteMsg=warning  WriteAfterWriteMsg=warning  WriteAfterReadMsg=warning  ShowAdditionalParam=off  OutDataTypeStr=uint8
  u8ModeCmd : DataStoreMemory  DataStoreName=u8ModeCmd  ReadBeforeWriteMsg=warning  WriteAfterWriteMsg=warning  WriteAfterReadMsg=warning  ShowAdditionalParam=off  OutDataTypeStr=uint8
  u8PriFutEnable : DataStoreMemory  DataStoreName=u8PriFutEnable  ReadBeforeWriteMsg=warning  WriteAfterWriteMsg=warning  WriteAfterReadMsg=warning  ShowAdditionalParam=off  OutDataTypeStr=uint8
  u8RdReqMsgPntr : DataStoreMemory  DataStoreName=u8RdReqMsgPntr  ReadBeforeWriteMsg=warning  WriteAfterWriteMsg=warning  WriteAfterReadMsg=warning  ShowAdditionalParam=off  OutDataTypeStr=uint8
  u8RedunModeCmd : DataStoreMemory  DataStoreName=u8RedunModeCmd  ReadBeforeWriteMsg=warning  WriteAfterWriteMsg=warning  WriteAfterReadMsg=warning  ShowAdditionalParam=off  OutDataTypeStr=uint8
  u8Reserved1 : DataStoreMemory  DataStoreName=u8Reserved1  ReadBeforeWriteMsg=warning  WriteAfterWriteMsg=warning  WriteAfterReadMsg=warning  ShowAdditionalParam=off  OutDataTypeStr=uint8
  u8SinglePhaseLeg : DataStoreMemory  DataStoreName=u8SinglePhaseLeg  ReadBeforeWriteMsg=warning  WriteAfterWriteMsg=warning  WriteAfterReadMsg=warning  ShowAdditionalParam=off  OutDataTypeStr=uint8
  u8TReserved1 : DataStoreMemory  DataStoreName=u8TReserved1  ReadBeforeWriteMsg=warning  WriteAfterWriteMsg=warning  WriteAfterReadMsg=warning  ShowAdditionalParam=off  OutDataTypeStr=uint8
  u8TclllcP1 : DataStoreMemory  DataStoreName=u8TclllcP1  ReadBeforeWriteMsg=warning  WriteAfterWriteMsg=warning  WriteAfterReadMsg=warning  ShowAdditionalParam=off  OutDataTypeStr=uint8
  u8TclllcP2 : DataStoreMemory  DataStoreName=u8TclllcP2  ReadBeforeWriteMsg=warning  WriteAfterWriteMsg=warning  WriteAfterReadMsg=warning  ShowAdditionalParam=off  OutDataTypeStr=uint8
  u8ThermalFlags : DataStoreMemory  DataStoreName=u8ThermalFlags  ReadBeforeWriteMsg=warning  WriteAfterWriteMsg=warning  WriteAfterReadMsg=warning  ShowAdditionalParam=off  OutDataTypeStr=uint8
  u8TnpcA : DataStoreMemory  DataStoreName=u8TnpcA  ReadBeforeWriteMsg=warning  WriteAfterWriteMsg=warning  WriteAfterReadMsg=warning  ShowAdditionalParam=off  OutDataTypeStr=uint8
  u8TnpcB : DataStoreMemory  DataStoreName=u8TnpcB  ReadBeforeWriteMsg=warning  WriteAfterWriteMsg=warning  WriteAfterReadMsg=warning  ShowAdditionalParam=off  OutDataTypeStr=uint8
  u8TnpcC : DataStoreMemory  DataStoreName=u8TnpcC  ReadBeforeWriteMsg=warning  WriteAfterWriteMsg=warning  WriteAfterReadMsg=warning  ShowAdditionalParam=off  OutDataTypeStr=uint8
  sim_cmp : Outport
  sim_va_seq : Outport  Port=2
  sim_vb_seq : Outport  Port=3
  sim_vc_seq : Outport  Port=4
  wires:
  sim_adc_quantized/1 -> CONTROL/1(adc_in)
  Demux/1 -> Variant Source/1
  CONTROL/1(sim_cmp) -> sim_cmp/1
  CONTROL/4(sim_vc_seq) -> sim_vc_seq/1
  CONTROL/2(sim_va_seq) -> sim_va_seq/1
  sim_adcinta/1 -> Variant Source/2
  Variant Source/1 -> CONTROL/Trigger
  CONTROL/3(sim_vb_seq) -> sim_vb_seq/1
  C28x Hardware Interrupt2/1 -> Demux/1
  Variant Source1/1 -> CANRX/Trigger
  Demux/2 -> Variant Source1/1
  Constant32/1 -> Vector Concatenate/4
  Constant1/1 -> Data Store Write/1
  Constant28/1 -> Data Store Write26/1
  Vector Concatenate/1 -> Data Store Write31/1
  Constant6/1 -> Data Store Write4/1
  Constant9/1 -> Data Store Write7/1
  Constant38/1 -> Data Store Write34/1
  Constant27/1 -> Data Store Write27/1
  Constant/1 -> Vector Concatenate/1
  Constant17/1 -> Data Store Write17/1
  Constant42/1 -> Data Store Write39/1
  Constant33/1 -> Vector Concatenate/2
  Constant4/1 -> Data Store Write2/1
  Constant12/1 -> Data Store Write11/1
  Constant26/1 -> Data Store Write25/1
  Constant40/1 -> Data Store Write37/1
  Constant35/1 -> Data Store Write32/1
  Constant3/1 -> Data Store Write1/1
  Constant29/1 -> Data Store Write28/1
  Constant18/1 -> Data Store Write14/1
  Constant36/1 -> Data Store Write36/1
  Constant14/1 -> Data Store Write8/1
  Constant41/1 -> Data Store Write38/1
  Constant31/1 -> Data Store Write29/1
  Constant5/1 -> Data Store Write3/1
  Constant11/1 -> Data Store Write10/1
  Constant37/1 -> Data Store Write33/1
  Constant16/1 -> Data Store Write15/1
  Constant13/1 -> Data Store Write16/1
  Constant39/1 -> Data Store Write35/1
  Constant8/1 -> Data Store Write6/1
  Constant34/1 -> Vector Concatenate/3
  Constant7/1 -> Data Store Write5/1
  Constant30/1 -> Data Store Write30/1
  Constant10/1 -> Data Store Write9/1

== system npc_controller/CANRX ==
  function : TriggerPort  TriggerType=function-call  VariantControl=Variant
  Function-Call Generator2 : simulink/Ports & Subsystems/Function-Call Generator  sample_time=-1  numberOfIterations=1  DisallowWideOutput=off
  can_rcv : Subsystem  TreatAsAtomicUnit=on
  wires:
  Function-Call Generator2/1 -> can_rcv/Trigger

== system npc_controller/CONTROL ==
  adc_in : Inport
  function : TriggerPort  TriggerType=function-call  VariantControl=Variant  PortDimensions=1
  CONTROL : Subsystem  TreatAsAtomicUnit=on
      settings: RTWSystemCode=Inline
  Constant : Constant  Commented=on  Value=V2G_en  OutDataTypeStr=single  SampleTime=-1
  Data Store Read : DataStoreRead  DataStoreName=control_en  IndexOptions=Index vector (dialog)  Indices=1  OutputSizes=1
  Data Store Read1 : DataStoreRead  DataStoreName=V2GCurTarget  IndexOptions=Index vector (dialog)  Indices=1  OutputSizes=1
  Data Store Write : DataStoreWrite  DataStoreName=control_en  IndexOptions=Index vector (dialog)  Indices=1  OutputSizes=1
  Data Store Write1 : DataStoreWrite  DataStoreName=burst_en  IndexOptions=Index vector (dialog)  Indices=1  OutputSizes=1
  Data Store Write2 : DataStoreWrite  DataStoreName=eoss  IndexOptions=Index vector (dialog)  Indices=1  OutputSizes=1
  Data Store Write3 : DataStoreWrite  DataStoreName=calib_ok  IndexOptions=Index vector (dialog)  Indices=1  OutputSizes=1
  Function-Call Generator : simulink/Ports & Subsystems/Function-Call Generator  sample_time=-1  numberOfIterations=1  DisallowWideOutput=off
  Function-Call Split{,1..4} (5 alike) : FunctionCallSplit  NumOutputPorts=2
  GET_ADC : Subsystem  TreatAsAtomicUnit=on  RTWFcnName=Cla1Task1  RTWFileName=sample_cla
      settings: RTWSystemCode=Inline  RTWFileNameOpts=User specified  RTWMemSecFuncInitTerm=Default  RTWMemSecFuncExecute=CpuToCla1MsgRAM  RTWMemSecDataInternal=Default
  GPIO_HIGH : Subsystem
      settings: RTWSystemCode=Inline
  GPIO_LOW : Subsystem
      settings: RTWSystemCode=Inline
  POLARITY : Subsystem  TreatAsAtomicUnit=on  RTWFcnName=Cla1Task1  RTWFileName=sample_cla
      settings: RTWSystemCode=Inline  RTWFileNameOpts=User specified  RTWMemSecFuncInitTerm=Default  RTWMemSecFuncExecute=CpuToCla1MsgRAM  RTWMemSecDataInternal=Default
  STATE-MACHINE : Subsystem
  SVPWM : Subsystem  Commented=on  TreatAsAtomicUnit=on
  Switch : Switch  Commented=on  Criteria=u2 > Threshold  SaturateOnIntegerOverflow=off  InputSameDT=off
  Variant Sink : VariantSink
  Variant Sink1 : VariantSink
  Variant Sink2 : VariantSink
  sim_cmp : Outport
  sim_va_seq : Outport  Port=2
  sim_vb_seq : Outport  Port=3
  sim_vc_seq : Outport  Port=4
  wires:
  GET_ADC/1(adc_out) -> STATE-MACHINE/1(adc_out), POLARITY/1(adc_in)
  adc_in/1 -> GET_ADC/1(adc_in)
  Function-Call Split/1 -> GET_ADC/Trigger
  Function-Call Generator/1 -> Function-Call Split2/1
  STATE-MACHINE/5(ref) -> Switch/3
  Function-Call Split3/1 -> STATE-MACHINE/Trigger
  Function-Call Split2/1 -> GPIO_HIGH/Trigger
  Function-Call Split2/2 -> Function-Call Split/1
  Function-Call Split1/1 -> CONTROL/Trigger
  Function-Call Split3/2 -> GPIO_LOW/Trigger
  Function-Call Split/2 -> Function-Call Split4/1
  Function-Call Split1/2 -> Function-Call Split3/1
  CONTROL/1(sim_cmp1) -> sim_cmp/1
  GET_ADC/2(adc_rect) -> CONTROL/1(adc_rect1)
  Variant Sink2/1 -> sim_vc_seq/1
  Variant Sink1/1 -> sim_va_seq/1
  STATE-MACHINE/11(vc_seq) -> Variant Sink2/1
  Variant Sink/1 -> sim_vb_seq/1
  STATE-MACHINE/9(va_seq) -> Variant Sink1/1
  STATE-MACHINE/10(vb_seq) -> Variant Sink/1
  STATE-MACHINE/3(burst_en) -> Data Store Write1/1
  Function-Call Split4/2 -> Function-Call Split1/1
  Function-Call Split4/1 -> POLARITY/Trigger
  POLARITY/1(pol_pha) -> CONTROL/5(pol_pha1)
  POLARITY/2(pol_phb) -> CONTROL/6(pol_phb1)
  POLARITY/3(pol_phc) -> CONTROL/7(pol_phc1)
  STATE-MACHINE/7(angle) -> CONTROL/4(angle1)
  STATE-MACHINE/1(calib_ok) -> Data Store Write3/1
  STATE-MACHINE/2(control_en) -> Data Store Write/1
  Data Store Read/1 -> CONTROL/2(control_en1)
  STATE-MACHINE/12(pha_en) -> CONTROL/8(pha_en1)
  STATE-MACHINE/13(phb_en) -> CONTROL/9(phb_en1)
  STATE-MACHINE/14(phc_en) -> CONTROL/10(phc_en1)
  CONTROL/2(Vpk) -> STATE-MACHINE/2(Vpk)
  STATE-MACHINE/4(eoss) -> Data Store Write2/1
  STATE-MACHINE/15(pfc_ok1) -> CONTROL/11(pfc_ok2)
  Constant/1 -> Switch/2
  Data Store Read1/1 -> CONTROL/3(ref1)

== system npc_controller/IDLE_AND_TIMER ==
  note: 1) Add Subsystem or Model blocks as valid variant choices.
      | 2) You cannot connect blocks at this level. At simulation, connectivity is automatically
      | determined, based on the active variant and port name matching.
  codegen : Subsystem  VariantControl=sim_en==false
  sim : Subsystem  VariantControl=sim_en==true

== system npc_controller/CANRX/can_rcv ==
  note: Read the CAN Data
  function : TriggerPort  TriggerType=function-call  VariantControl=Variant
  Bitwise AND : simulink/Logic and Bit Operations/Bitwise Operator  logicop=AND  UseBitMask=on  BitMask=hex2dec('0000003F')  BitMaskRealWorld=Stored Integer
  CANA_CAN0INT : idelinklib_common/Memory Copy  Priority=2  copyFrom=Specified source code symbol  copyFromAddressSource=Specify via dialog  copyFromAddress=hex2dec('48108')  copyFromSrcCode=(CANA_BASE + CAN_O_INT)  dataTypeFrom=uint32  dataDimensionFrom=1  useOffsetFrom=off  offsetFromSrc=Specify via dialog  offsetFrom=0  strideFrom=1  copyTo=Output port  copyToAddressSource=Specify via dialog  copyToAddress=hex2dec('00002000')  copyToSrcCode=myVariableDst  dataTypeTo=uint32  useOffsetTo=off  offsetToSrc=Specify via dialog  offsetTo=0  strideTo=1  sampleTime=-1  useInitValue=off  initValueSrc=Specify constant value  initValue=1  initValueSrcCode=myInitValueVariable  useAsMask=off  maskOperator=bitwise AND  useTermValue=off  termValue=1  isRealtimeEnabled=off  emitCCBeforeWrite=off  CCBeforeWrite=/* Custom Code Before Write*/  emitCCAfterWrite=off  CCAfterWrite=/* Custom Code After Write*/  useDMACopy=off  enableBlockingMode=off
      settings: SourceProductBaseCode=ME
  Constant : Constant  Commented=on
  Digital Output : c2837xDlib/Digital Output  Commented=on  GPIO_Number=GPIO8~GPIO15  GPIO_Bit0=off  GPIO_BIT0_Toggle=off  GPIO_Bit1=off  GPIO_BIT1_Toggle=off  GPIO_Bit2=off  GPIO_BIT2_Toggle=off  GPIO_Bit3=off  GPIO_BIT3_Toggle=off  GPIO_Bit4=off  GPIO_BIT4_Toggle=off  GPIO_Bit5=on  GPIO_BIT5_Toggle=on  GPIO_Bit6=off  GPIO_BIT6_Toggle=off  GPIO_Bit7=off  GPIO_BIT7_Toggle=off
      settings: SourceProductBaseCode=TIC2000
  Switch Case : SwitchCase  CaseConditions={10,11,12}  ShowDefaultCase=off
  Switch Case Action Subsystem : Subsystem  TreatAsAtomicUnit=on
  Switch Case Action Subsystem1 : Subsystem  TreatAsAtomicUnit=on
  Switch Case Action Subsystem2 : Subsystem  TreatAsAtomicUnit=on
  wires:
  Switch Case/1 -> Switch Case Action Subsystem/Action
  Switch Case/3 -> Switch Case Action Subsystem2/Action
  Switch Case/2 -> Switch Case Action Subsystem1/Action
  CANA_CAN0INT/1 -> Bitwise AND/1
  Bitwise AND/1 -> Switch Case/1
  Constant/1 -> Digital Output/1
